simulink model "RT_IGBT"  (R2024b)
settings: Solver=ode4  StartTime=0.0  StopTime=2  FixedStep=Ts  RelTol=1e-3
PreLoadFcn:
  | Net_improve_init;L=Lac_MV;Tctrl=Ts;
PostLoadFcn:
  | Net_improve_init;L=Lac_MV;Tctrl=Ts;
InitFcn:
  | Net_improve_init;L=Lac_MV;Tctrl=Ts;
undefined symbols (not defined in the file): C1, dend, DiscIntNeverNeededParam, f_cari, fs, Lac_MV, numd, Pref, R1, Rac_MV, Ts, Vac_peak_MV, Vdc
libraries: powerlib_extras x5, spsControlledVoltageSourceLib x4, artemis x3, spsCurrentMeasurementLib x3, spsSeriesRLCBranchLib x3, spsVoltageMeasurementLib x3, rtlab x2, spsThreePhaseVIMeasurementLib x2, spsGroundLib x2, spsUniversalBridgeLib x1, spsIdealSwitchLib x1, spsPower3phInstantaneousLib x1
Description:
  | The Model initialization function Callback automatically
  | 
  | sets the sample time  to 2e-6 sec.  and loads the initial
  | 
  | states vector xInitial. The initial state vector is saved in the
  | 
  | power_acdrive_init.mat file.
  | 
  | 
  | 
  | Check  the Initial state checkbox in the Simulation
  | 
  | parameters/Workspace I/O to start in steady state with a
  | 
  | speed of 120 rad/s and a torque of 0 N.m/s,
  | 
  | 
  | Copyright 2008-2015 The MathWorks, Inc.
settings Model: Creator=WeiLi  LastModifiedBy=KeXing
settings SolverCC: AlgebraicLoopSolver=TrustRegion
settings DataIOCC: SaveFinalState=on  SaveFormat=Array  SignalLoggingSaveFormat=ModelDataLogs  SaveOutput=off  SaveTime=off  ReturnWorkspaceOutputs=off  SignalLoggingName=sigsOut
settings OptimizationCC: BlockReduction=off  ExpressionDepthLimit=2147483647  InitFltsAndDblsToZero=on  LifeSpan=inf
settings DebuggingCC: SaveWithParameterizedLinksMsg=none  UnderspecifiedInitializationDetection=Classic  MergeDetectMultiDrivingBlocksExec=none  CheckExecutionContextPreStartOutputMsg=on  SignalResolutionControl=TryResolveAllWithWarning  MultiTaskDSMMsg=warning  MultiTaskCondExecSysMsg=none  FcnCallInpInsideContextMsg=warning  UnconnectedInputMsg=warning  UnconnectedLineMsg=warning  StateNameClashWarn=warning  SFUnexpectedBacktrackingDiag=warning  SFNoUnconditionalDefaultTransitionDiag=warning  SFExecutionAtInitializationDiag=none  ArithmeticOperatorsInVariantConditions=warning
settings HardwareCC: ProdBitPerPointer=32  ProdBitPerSizeT=32  ProdBitPerPtrDiffT=32  ProdLargestAtomicFloat=None  ProdIntDivRoundTo=Undefined  ProdEndianess=Unspecified  ProdWordSize=32  ProdHWDeviceType=32-bit Generic  TargetUnknown=on
settings ModelReferenceCC: EnableRefExpFcnMdlSchedulingChecks=on  PropagateSignalLabelsOutOfModel=off
settings SFSimCC: SimUseLocalCustomCode=off  CustomCodeUndefinedFunction=UseInterfaceOnly
settings RTWCC: RTWUseLocalCustomCode=off  GPUComputeCapability=3.5
settings CodeAppCC: StateflowObjectComments=on
settings GRTTargetCC: TargetFcnLib=ansi_tfl_tmw.mat  TargetLangStandard=C89/C90 (ANSI)  CombineOutputUpdateFcns=off  GRTInterface=on
settings ConfigComp: CovMetricSettings=dw  CovSaveCumulativeToWorkspaceVar=on  CovSaveSingleToWorkspaceVar=on  CovExternalEMLEnable=off
settings SimscapeCC: SimscapeNormalizeSystem=off

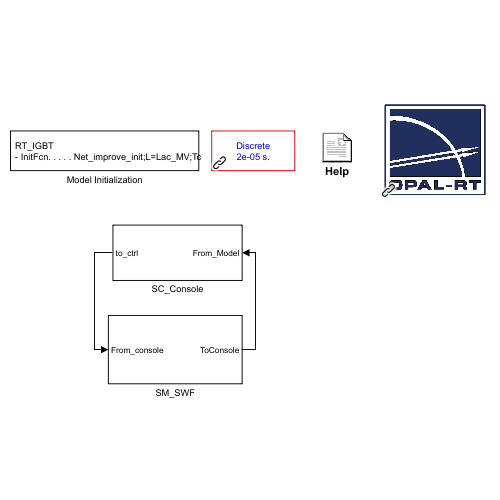
[thumbnail: Simulink's stored preview of the top-level diagram]
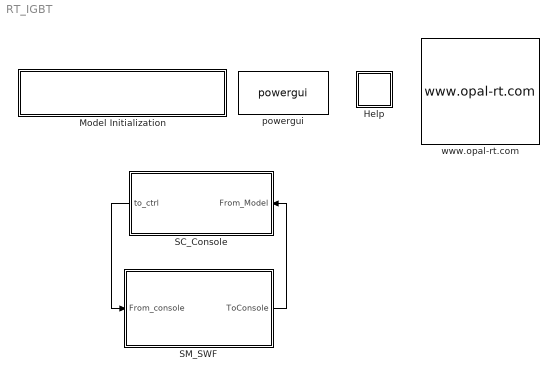
== system RT_IGBT ==
  Help : Subsystem  mask(OpDoc){docfile=../Help/help.html}
      mask init:
      | %patch([1,1,0,0,.8,1],[.8,0,0,1,1,.8],[.8 .8 .8]);
      | %patch([.15 .78 .78 .15 .15],[.8 .8 .83 .83 .8],[.9 .9 .9]);
      | %patch([.15 .78 .78 .15 .15],[.7 .7 .73 .73 .8],[.9 .9 .9]);
      | %patch([.15 .78 .78 .15 .15],[.6 .6 .63 .63 .6],[.9 .9 .9]);
      | %patch([.15 .78 .78 .15 .15],[.5 .5 .53 .53 .5],[.9 .9 .9]);
      | %patch([.15 .78 .78 .15 .15],[.4 .4 .43 .43 .4],[.9 .9 .9]);
      settings: OpenFcn=OpHelp_cb(gcb);
      mask Display: image(imread('opdoc.bmp'))
  Model Initialization : Subsystem  mask(Model Functions){InitFcnX=Net_improve_init;L=Lac_MV;Tctrl=Ts;, prel=on, posl=on, inif=on, strf=off}
      mask prompts: InitFcnX "Initialisation"; prel "Preload Function"; posl "PostLoad Function"; inif "InitFcn"; strf "StartFcn"
      mask init:
      | currentBlock = gcb;
      | root = bdroot(currentBlock);
      | 
      | if ~strcmp(get_param(root,'BlockDiagramType'),'library')
      |     if prel==1
      |         set_param(root, 'PreLoadFcn', InitFcnX);
      |     else
      |         set_param(root, 'PreLoadFcn', '');
      |     end
      |     if inif==1
      |         set_param(root, 'InitFcn', InitFcnX);
      |     else
      |         set_param(root, 'InitFcn', '');
      |     end
      |     if strf==1
      |         set_param(root, 'StartFcn', InitFcnX);
      |     else
      |         set_param(root, 'StartFcn', '');
      |     end
      |     if posl==1
      |         set_param(root, 'PostLoadFcn', InitFcnX);
      |     else
      |         set_param(root, 'PostLoadFcn', '');
      |     end
      | end
      | 
      | pos = get_param(currentBlock, 'Position');
      | width = pos(3) - pos(1); height = pos(4) - pos(2);
      | txt = [ upper(root) '\n' '- InitFcn. . . . . '  get_param(root, 'InitFcn') ];
      settings: CopyFcn=set_param(gcb,'LinkStatus','none')
      mask Display: text(5, height*0.5, txt, 'horizontalAlignment', 'left', 'verticalAlignment', 'middle') ;
  SC_Console : Subsystem
  SM_SWF : Subsystem
  powergui : spspowerguiLib/powergui  Priority=2  SimulationMode=Discrete  SampleTime=Ts  frequency=60  Iterations=50  frequencyindice=0  Pbase=100e6  ErrMax=1e-4  UnitsV=kV  UnitsW=MW  buscounter=0  FunctionMessages=off  echomessages=off  EnableUseOfTLC=off  CurrentSourceSwitches=off  DisableSnubberDevices=off  DisableRonSwitches=off  DisableVfSwitches=off  DisplayEquations=off  AutomaticDiscreteSolvers=off  SolverType=Backward Euler  Interpol=off  ExternalGateDelay=off  methode=off  Ts=0  x0status=blocks  SPID=off  SwTol=0  HookPort=off  NonlinearTolerance=1e-4  nMaxIteration=100  ContinueOnMaxIteration=off  RestoreLinks=warning  ResistiveCurrentMeasurement=off  Frange=[0:2:500]  Ylog=off  Xlog=on  ShowGrid=off  save=off  variable=ZData  structure=VI  ZoomFFT=off  StartTime=9  cycles=10  DisplayStyle=2  fundamental=300/pi  FreqAxis=off  MaxFrequency=1000  frequencyindicesteady=1  RmsSteady=1  display=off
  www.opal-rt.com : artemis/Internal/www.opal-rt.com  SystemSampleTime=-1  VariantActivationTime=update diagram  AllowFlexibleInterface=on  Latency=0  AutoFrameSizeCalculation=off
      settings: SourceProductName=Artemis
  wires:
  SM_SWF/1(ToConsole) -> SC_Console/1(From_Model)
  SC_Console/1(to_ctrl) -> SM_SWF/1(From_console)

== system RT_IGBT/Help ==

== system RT_IGBT/Model Initialization ==

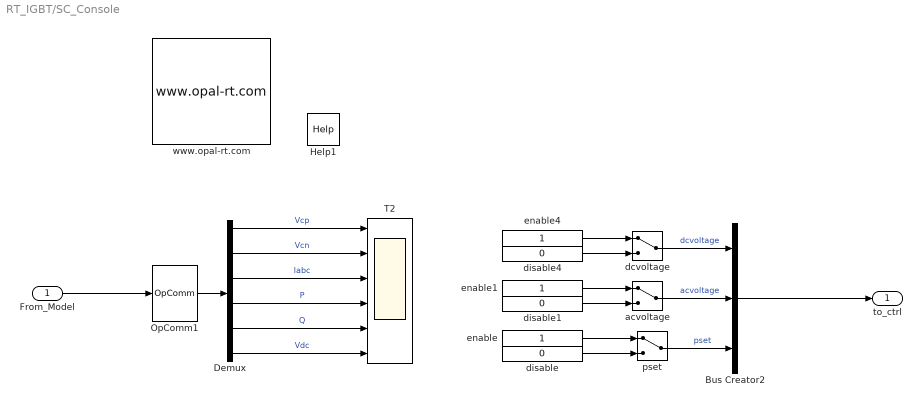
== system RT_IGBT/SC_Console ==
  From_Model : Inport
  Bus Creator2 : BusCreator  Inputs=3
  Demux : Demux  Outputs=6
  Help1 : artemis/Internal/Help  docfile=../help/help.html
      settings: SourceProductName=Artemis
  OpComm1 : rtlab/OpComm  nbport=1  groupe_acq=1  subsys_rate=Ts  st=0  Synchronization=off  Interpolation=on  Threshold=1.0  Missed_Data=off  Sim_Time=off  Samples=off  dynSigOut=off  from_console=0  warning_done=off  writeOpCommFile=off  Offset=off
      settings: SourceProductName=RT-LAB
  T2 : Scope  NumInputPorts=6
  acvoltage : ManualSwitch
  dcvoltage : ManualSwitch
  disable : Constant  Value=0
  disable1 : Constant  Value=0
  disable4 : Constant  Value=0
  enable : Constant
  enable1 : Constant
  enable4 : Constant
  pset : ManualSwitch
  www.opal-rt.com : artemis/Internal/www.opal-rt.com  SystemSampleTime=-1  VariantActivationTime=update diagram  AllowFlexibleInterface=on  Latency=0  AutoFrameSizeCalculation=off
      settings: SourceProductName=Artemis
  to_ctrl : Outport
  wires:
  enable/1 -> pset/1
  Demux/2 -> T2/2  "Vcn"
  OpComm1/1 -> Demux/1
  Bus Creator2/1 -> to_ctrl/1
  From_Model/1 -> OpComm1/1
  Demux/4 -> T2/4  "P"
  Demux/1 -> T2/1  "Vcp"
  acvoltage/1 -> Bus Creator2/2  "acvoltage"
  disable1/1 -> acvoltage/2
  disable/1 -> pset/2
  enable1/1 -> acvoltage/1
  Demux/3 -> T2/3  "Iabc"
  disable4/1 -> dcvoltage/2
  enable4/1 -> dcvoltage/1
  dcvoltage/1 -> Bus Creator2/1  "dcvoltage"
  pset/1 -> Bus Creator2/3  "pset"
  Demux/5 -> T2/5  "Q"
  Demux/6 -> T2/6  "Vdc"

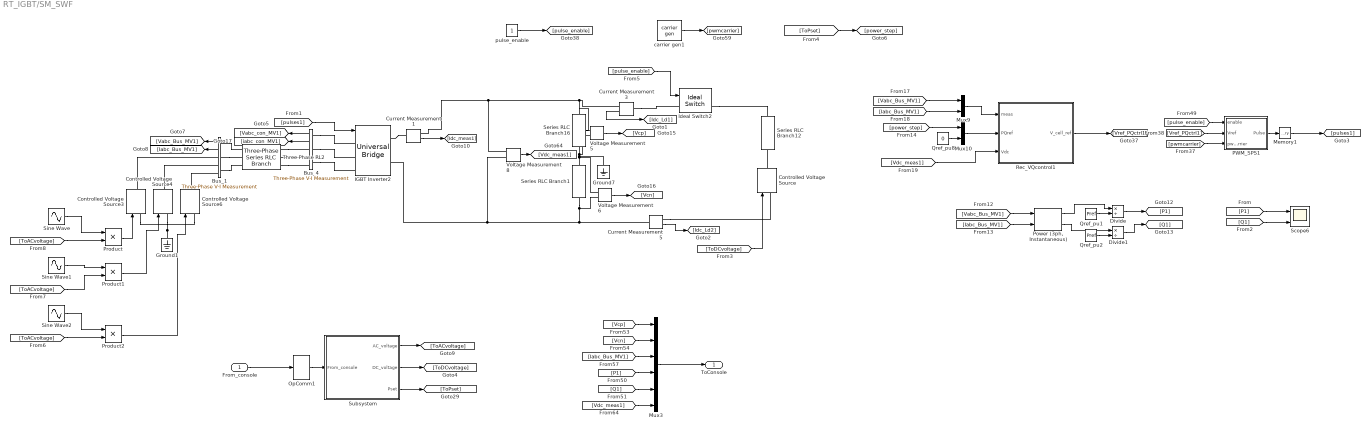
== system RT_IGBT/SM_SWF ==
  From_console : Inport
  Bus_1 : spsThreePhaseVIMeasurementLib/Three-Phase V-I Measurement  VoltageMeasurement=phase-to-ground  SetLabelV=off  LabelV=Vabc  Vpu=off  VpuLL=off  CurrentMeasurement=yes  SetLabelI=off  LabelI=Iabc  Ipu=off  Pbase=P_AC  Vbase=V_AC_prim  OutputType=Complex  PhasorSimulation=off  PSBequivalent=0
  Bus_4 : spsThreePhaseVIMeasurementLib/Three-Phase V-I Measurement  VoltageMeasurement=phase-to-ground  SetLabelV=off  LabelV=Vabc  Vpu=off  VpuLL=off  CurrentMeasurement=yes  SetLabelI=off  LabelI=Iabc  Ipu=off  Pbase=P_AC  Vbase=V_AC_prim  OutputType=Complex  PhasorSimulation=off  PSBequivalent=0
  Controlled Voltage Source : spsControlledVoltageSourceLib/Controlled Voltage Source  Initialize=on  Source_Type=DC  Amplitude=3000  Phase=0  Frequency=0  Measurements=None
  Controlled Voltage Source3 : spsControlledVoltageSourceLib/Controlled Voltage Source  Initialize=off  Source_Type=AC  Amplitude=0  Phase=0  Frequency=fs  Measurements=None
  Controlled Voltage Source4 : spsControlledVoltageSourceLib/Controlled Voltage Source  Initialize=off  Source_Type=AC  Amplitude=0  Phase=0  Frequency=fs  Measurements=None
  Controlled Voltage Source6 : spsControlledVoltageSourceLib/Controlled Voltage Source  Initialize=off  Source_Type=AC  Amplitude=0  Phase=0  Frequency=fs  Measurements=None
  Current Measurement1 : spsCurrentMeasurementLib/Current Measurement  PhasorSimulation=off  OutputType=Complex  PSBequivalent=0
  Current Measurement3 : spsCurrentMeasurementLib/Current Measurement  PhasorSimulation=off  OutputType=Complex  PSBequivalent=0
  Current Measurement5 : spsCurrentMeasurementLib/Current Measurement  PhasorSimulation=off  OutputType=Complex  PSBequivalent=0
  Divide : Product  Inputs=*/
  Divide1 : Product  Inputs=*/
  Ground1 : spsGroundLib/Ground  LConnTagsString=a
  Ground7 : spsGroundLib/Ground  LConnTagsString=a
  IGBT Inverter2 : spsUniversalBridgeLib/Universal Bridge  Arms=3  SnubberResistance=IGBT_Rs  SnubberCapacitance=1e-6  Device=IGBT / Diodes  Ron=IGBT_Ron  Lon=0  ForwardVoltages=[0 0]  ForwardVoltage=.8  GTOparameters=[ 1e-6 , 1e-6 ]  IGBTparameters=[0 0]  Measurements=Device voltages  Measurements_2=None  converterType=Rectifier
      settings: AttributesFormatString=\n
  Ideal Switch2 : spsIdealSwitchLib/Ideal Switch  Ron=0.001  Lon=0  IC=0  Rs=1e9  Cs=inf  Measurements=on
  Memory1 : Memory
  Mux10 : Mux  Inputs=2
  Mux3 : Mux  Inputs=6
  Mux9 : Mux  Inputs=2
  OpComm1 : rtlab/OpComm  nbport=1  groupe_acq=1  subsys_rate=Ts  st=0  Synchronization=on  Interpolation=on  Threshold=1.0  Missed_Data=off  Sim_Time=off  Samples=off  dynSigOut=off  from_console=1  warning_done=off  writeOpCommFile=off  Offset=off
      settings: SourceProductName=RT-LAB
  PWM_SPS1 : Subsystem
  "Power (3ph, Instantaneous)" : spsPower3phInstantaneousLib/Power (3ph, Instantaneous)
  Product : Product
  Product1 : Product
  Product2 : Product
  Qref_pu1 : Constant  Value=Pref
  Qref_pu2 : Constant  Value=Pref
  Qref_pu8 : Constant  Value=0
  Rec_VQcontrol1 : Subsystem  mask(converter controller){cm=off, base=[Pref, Vac_peak_MV*sqrt(3/2), Vdc/2, fs], LRx=[Lac_MV, Rac_MV], LRx_inpu=off, Kd=[0.3  2]*10/6  %was [1 0.1]   ; [0.1  1]*1, Kp=[0.3 1]*1     %was [1 0.1]   ; [0.1  1]*1, Kvdc=[2 10]*1;   %was [0.5 1]*20 for Cdc=320uF, Vabc_lim=[-1 1], limitVdq=1.1, nadv=6, xtrIctrl1=[0.4 10 10 -10], Ts=Tctrl}
      mask prompts: cm "control mode (check VQ/uncheck PQ), only one terminal in VQ mode"; base "base value for power(VA), ac voltage(V), dc voltage to ground(V), and frequenvy(Hz) [Sb, Vb, Vdcb,freq]"; LRx "commutation inductance and resistance [Lx, Rx]"; LRx_inpu "[Lx, Rx] in pu if checked/ SI unchecked"; Kd "Kp Ki for d-axis PI control [kp ki]"; Kp "Kp Ki for q-axis PI control [kp ki]"; Kvdc "Kp Ki for Vdc PI control [kp ki]"; Vabc_lim "output Vabc limit [min max]"; limitVdq "limit for Vd,Vq (pu, default = 1.1)"; nadv "nb of time step to compesate for delay (default=1)"; xtrIctrl1 "[kp, kp, limitmax, limitmin] for current control (default=[0.4, 10, 10, -10])"
      mask help:
      | input 1, 6 dimentions, Vabc, Iabc, (SI)
      | input 2, 2 dimentions, Pref, Qref (PU)
      | input 3, 6 dimentions, Vcap at up arm a, lower arm a, up arm b, lower arm b, up arm c and lower arm c.
      | input 4, 1 dimention, pulse on
      | input 5, 1 dimention
      |
      | power or current directions: to go into grid is positive
      mask init:
      | if cm==0;
      |     x=['PQ\nmode'];
      | else
      |     x=['VQ\nmode'];
      | end
      | 
      | Sb=base(1);            %VA 3phase power base;
      | Vb=base(2);       %V, line-line rms voltage base
      | Ib=Sb/(sqrt(3)*Vb); %A, rms current base
      | Zb=Vb^2/Sb ;        %ohm, impedence base
      | Vdc=base(3);      %V Vdc+ to ground or ground to Vdc- 
      | frq=base(4);
      | 
      | if LRx_inpu
      |     Rxpu=LRx(2);
      |     Lxpu=LRx(1);
      | else
      |     Rxpu=LRx(2)/Zb;
      |     Lxpu=LRx(1)*2*pi*frq/Zb;
      | end;
      | 
      | ks=Vdc*sqrt(3/2)/Vb;     % ma=1/ks for 1pu dc ->1pu ac;
      | 
      | Kp=Kd;
      mask DialogControl ParameterTabVar0 Prompt: parameters
      mask DialogControl ParameterTabVar01 Prompt: advanced
      mask Display: disp (x);
  Scope6 : Scope  NumInputPorts=2
  Series RLC Branch1 : spsSeriesRLCBranchLib/Series RLC Branch  LConnTagsString=__new0  RConnTagsString=__new0  BranchType=C  Resistance=R1  Inductance=1e-3  SetiL0=off  InitialCurrent=0  Capacitance=C1  Setx0=off  InitialVoltage=0  Measurements=None
  Series RLC Branch12 : spsSeriesRLCBranchLib/Series RLC Branch  LConnTagsString=__new0  RConnTagsString=__new0  BranchType=R  Resistance=3e3^2/(Pref)/10*2  Inductance=1e-3  SetiL0=off  InitialCurrent=0  Capacitance=C1  Setx0=off  InitialVoltage=0  Measurements=None
  Series RLC Branch16 : spsSeriesRLCBranchLib/Series RLC Branch  LConnTagsString=__new0  RConnTagsString=__new0  BranchType=C  Resistance=R1  Inductance=1e-3  SetiL0=off  InitialCurrent=0  Capacitance=C1  Setx0=off  InitialVoltage=0  Measurements=None
  Sine Wave : Sin  Amplitude=3e3/2*sqrt(2/3)  Frequency=2*pi*fs  SampleTime=0
  Sine Wave1 : Sin  Amplitude=3e3/2*sqrt(2/3)  Frequency=2*pi*fs  Phase=-2*pi/3  SampleTime=0
  Sine Wave2 : Sin  Amplitude=3e3/2*sqrt(2/3)  Frequency=2*pi*fs  Phase=+2*pi/3  SampleTime=0
  Subsystem : Subsystem
  Three-Phase RL2 : spsThreePhaseSeriesRLCBranchLib/Three-Phase Series RLC Branch  LConnTagsString=A|B|C  RConnTagsString=A|B|C  BranchType=RL  Resistance=Rac_MV  Inductance=Lac_MV  Capacitance=1e-6  Measurements=None
  Voltage Measurement5 : spsVoltageMeasurementLib/Voltage Measurement  PhasorSimulation=off  OutputType=Complex  PSBequivalent=0
  Voltage Measurement6 : spsVoltageMeasurementLib/Voltage Measurement  PhasorSimulation=off  OutputType=Complex  PSBequivalent=0
  Voltage Measurement8 : spsVoltageMeasurementLib/Voltage Measurement  PhasorSimulation=off  OutputType=Complex  PSBequivalent=0
  carrier gen1 : libMMCcpuv2/carrier gen  fc=f_cari*2  range=[ 1 -1]  Ms=3  Ns=1
  pulse_enable : Constant
  ToConsole : Outport
  wires:
  Bus_1/1 -> [Vabc_Bus_MV1]
  Subsystem/2(DC_voltage) -> [ToDCvoltage]
  Sine Wave1/1 -> Product1/1
  Bus_1/2 -> [Iabc_Bus_MV1]
  [Q1] -> Scope6/2
  Qref_pu2/1 -> Divide1/2
  From_console/1 -> OpComm1/1
  Product/1 -> Controlled Voltage Source3/1
  [pwmcarrier] -> PWM_SPS1/3(pwmcarrier)
  Bus_4/1 -> [Vabc_con_MV1]
  [pulse_enable] -> Ideal Switch2/1
  Mux3/1 -> ToConsole/1
  Divide1/1 -> [Q1]
  Voltage Measurement5/1 -> [Vcp]
  [Vabc_Bus_MV1] -> Mux9/1
  [P1] -> Mux3/4
  [Vcn] -> Mux3/2
  [pulses1] -> IGBT Inverter2/1
  Current Measurement5/1 -> [Idc_Ld2]
  Mux10/1 -> Rec_VQcontrol1/2(PQref)
  Sine Wave2/1 -> Product2/1
  [Q1] -> Mux3/5
  Bus_4/2 -> [iabc_con_MV1]
  Mux9/1 -> Rec_VQcontrol1/1(meas)
  OpComm1/1 -> Subsystem/1(From_console)
  [ToPset] -> [power_step]
  [ToACvoltage] -> Product/2
  Qref_pu8/1 -> Mux10/2
  Product2/1 -> Controlled Voltage Source6/1
  Subsystem/3(Pset) -> [ToPset]
  [power_step] -> Mux10/1
  pulse_enable/1 -> [pulse_enable]
  [Iabc_Bus_MV1] -> "Power (3ph, Instantaneous)"/2
  [ToDCvoltage] -> Controlled Voltage Source/1
  Current Measurement3/1 -> [Idc_Ld1]
  "Power (3ph, Instantaneous)"/2 -> Divide1/1
  Sine Wave/1 -> Product/1
  "Power (3ph, Instantaneous)"/1 -> Divide/1
  PWM_SPS1/1(Pulse) -> Memory1/1
  [Iabc_Bus_MV1] -> Mux9/2
  [Vabc_Bus_MV1] -> "Power (3ph, Instantaneous)"/1
  Voltage Measurement6/1 -> [Vcn]
  [Vdc_meas1] -> Mux3/6
  Qref_pu1/1 -> Divide/2
  Divide/1 -> [P1]
  Voltage Measurement8/1 -> [Vdc_meas1]
  [Vdc_meas1] -> Rec_VQcontrol1/3(Vdc)
  Memory1/1 -> [pulses1]
  [Vref_PQctrl1] -> PWM_SPS1/2(Vref)
  [Iabc_Bus_MV1] -> Mux3/3
  carrier gen1/1 -> [pwmcarrier]
  Rec_VQcontrol1/1(V_cell_ref) -> [Vref_PQctrl1]
  [P1] -> Scope6/1
  Current Measurement1/1 -> [Idc_meas1]
  [Vcp] -> Mux3/1
  Product1/1 -> Controlled Voltage Source4/1
  [pulse_enable] -> PWM_SPS1/1(enable)
  [ToACvoltage] -> Product2/2
  Subsystem/1(AC_voltage) -> [ToACvoltage]
  [ToACvoltage] -> Product1/2
  connections:
  Series RLC Branch1/LConn1 -- Voltage Measurement6/LConn1 -- Ground7/LConn1 -- Voltage Measurement5/LConn2 -- Series RLC Branch16/RConn1
  Controlled Voltage Source/RConn1 -- Series RLC Branch12/LConn1
  Bus_1/LConn2 -- Three-Phase RL2/LConn2
  Ground1/LConn1 -- Controlled Voltage Source6/LConn1 -- Controlled Voltage Source3/LConn1 -- Controlled Voltage Source4/LConn1
  Ideal Switch2/RConn1 -- Series RLC Branch12/RConn1
  Bus_4/LConn3 -- IGBT Inverter2/LConn3
  Series RLC Branch1/RConn1 -- Voltage Measurement6/LConn2 -- IGBT Inverter2/RConn2 -- Voltage Measurement8/LConn2 -- Current Measurement5/LConn1
  Three-Phase RL2/RConn1 -- Bus_4/RConn1
  Bus_1/LConn3 -- Three-Phase RL2/LConn3
  Voltage Measurement8/LConn1 -- Voltage Measurement5/LConn1 -- Series RLC Branch16/LConn1 -- Current Measurement3/RConn1 -- Current Measurement1/RConn1
  Current Measurement5/RConn1 -- Controlled Voltage Source/LConn1
  Three-Phase RL2/RConn3 -- Bus_4/RConn3
  Controlled Voltage Source4/RConn1 -- Bus_1/RConn2
  Bus_4/LConn2 -- IGBT Inverter2/LConn2
  Bus_1/LConn1 -- Three-Phase RL2/LConn1
  Current Measurement3/LConn1 -- Ideal Switch2/LConn1
  Three-Phase RL2/RConn2 -- Bus_4/RConn2
  Controlled Voltage Source3/RConn1 -- Bus_1/RConn1
  Current Measurement1/LConn1 -- IGBT Inverter2/RConn1
  Controlled Voltage Source6/RConn1 -- Bus_1/RConn3
  Bus_4/LConn1 -- IGBT Inverter2/LConn1

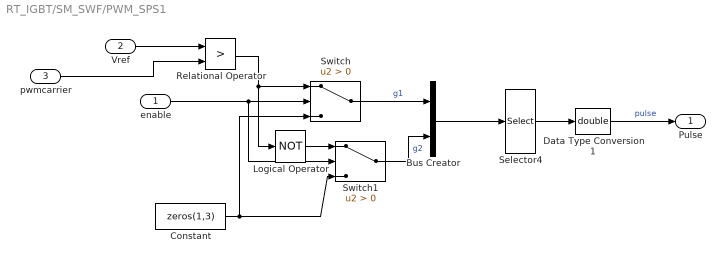
== system RT_IGBT/SM_SWF/PWM_SPS1 ==
  enable : Inport
  Vref : Inport  Port=2
  pwmcarrier : Inport  Port=3
  Bus Creator : BusCreator  Inputs=2
  Constant : Constant  Value=zeros(1,3)
  Data Type Conversion1 : DataTypeConversion  OutDataTypeStr=double  SaturateOnIntegerOverflow=off  RndMeth=Floor
  Logical Operator : Logic  Operator=NOT  AllPortsSameDT=off  OutDataTypeStr=boolean
  Relational Operator : RelationalOperator  Operator=>  OutDataTypeStr=boolean  InputSameDT=off
  Selector4 : Selector  InputPortWidth=6  IndexOptions=Index vector (dialog)  Indices=[1 4 2 5 3 6]  OutputSizes=1
  Switch : Switch  Criteria=u2 > Threshold  SaturateOnIntegerOverflow=off  InputSameDT=off
  Switch1 : Switch  Criteria=u2 > Threshold  SaturateOnIntegerOverflow=off  InputSameDT=off
  Pulse : Outport  VectorParamsAs1DForOutWhenUnconnected=off
  wires:
  Vref/1 -> Relational Operator/1
  pwmcarrier/1 -> Relational Operator/2
  enable/1 -> Switch1/2, Switch/2
  Relational Operator/1 -> Logical Operator/1, Switch/1
  Switch/1 -> Bus Creator/1  "g1"
  Switch1/1 -> Bus Creator/2  "g2"
  Logical Operator/1 -> Switch1/1
  Constant/1 -> Switch/3, Switch1/3
  Selector4/1 -> Data Type Conversion1/1
  Bus Creator/1 -> Selector4/1
  Data Type Conversion1/1 -> Pulse/1  "pulse"

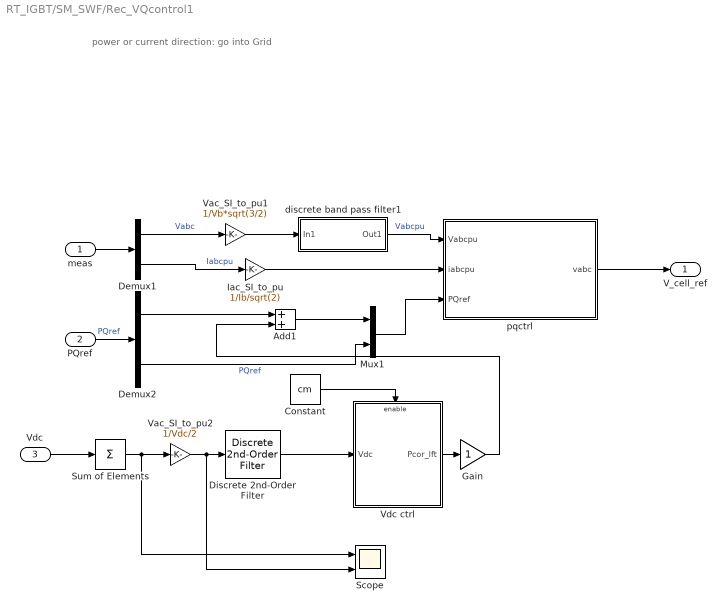
== system RT_IGBT/SM_SWF/Rec_VQcontrol1 ==
  note: power or current direction: go into Grid
  meas : Inport
  PQref : Inport  Port=2
  Vdc : Inport  Port=3
  Add1 : Sum
  Constant : Constant  Value=cm
  Demux1 : Demux  Outputs=[3 3 ]
  Demux2 : Demux  Outputs=2
  Discrete 2nd-Order Filter : powerlib_extras/Discrete  Control Blocks/Discrete  2nd-Order Filter  FilterType=Lowpass  Fo=90  Zeta=0.707  Ts=Ts  Initialize=off  Vac_Init=[0.8 -25 60]  Vdc_Init=-0.4  PlotResponse=off  param1=[1 500 1]
  Gain : Gain
  Iac_SI_to_pu : Gain  Gain=1/Ib/sqrt(2)
  Mux1 : Mux  Inputs=2
  Scope : Scope  NumInputPorts=2
  Sum of Elements : Sum  Inputs=+
  Vac_SI_to_pu1 : Gain  Gain=1/Vb*sqrt(3/2)
  Vac_SI_to_pu2 : Gain  Gain=1/Vdc/2  SampleTime=Ts
  Vdc ctrl : Subsystem
  discrete band pass filter1 : Subsystem  mask(discrete transfer Fcn generator){Fo=frq, adj1=1, inistate=0, Ts=Ts, bodedw=off}
      mask prompts: Fo "F0 (Hz)"; adj1 "adj (1 for no adjustment, larger adj for wider band pass)"; inistate "Initial states"; Ts "Sample time (must be explicite)"; bodedw "draw Bode diagram of filter"
      mask help:
      | This block transfer a continous TF to a discrete TF
      | using Bilinear (Tustin) approximation
      mask init:
      | AD1=tf([1 0],1);
      | 
      | %second order
      | % Fo=50; %cut off freq.
      | % omega0=Fo*2*pi;
      | % adj1=3;   %adjustment 1
      | Zeta= 0.707*adj1; %Damping factor Zeta ( Q = 1 / (2*Zeta) ):
      | Wo=2*pi*Fo;
      | % str=sprintf(' Fo=%iHz\n\n',Fo);
      |  n2=0; n1=0;n0=Wo*Wo;
      |  d2=1;d1=2*Zeta*Wo;d0=Wo*Wo;
      | numc=[n2 n1 n0];
      | denc=[d2 d1 d0];
      | AD3=tf(numc,denc);
      | 
      | AD4=AD1*AD3;
      | [mag1,pha1]=bode(AD4,Wo);
      | mag0=mag1;
      | AD=AD4/mag0;
      | 
      | if bodedw==1
      |     figure;
      |     h=bodeplot(AD1,AD3,AD);
      |     setoptions(h,'FreqUnits','Hz');
      |     grid on;
      |     title(['Bode Diagram, adj=',num2str(adj1)]);
      | end;
      |     
      | % gg=tf(num,den);
      | ggd=c2d(AD,Ts,'tustin');
      | [numd,dend] = tfdata(ggd,'v');
  pqctrl : Subsystem
  V_cell_ref : Outport  VectorParamsAs1DForOutWhenUnconnected=off
  wires:
  Constant/1 -> Vdc ctrl/Enable
  Vac_SI_to_pu1/1 -> discrete band pass filter1/1(In1)
  Vac_SI_to_pu2/1 -> Scope/2, Discrete 2nd-Order Filter/1
  Vdc/1 -> Sum of Elements/1
  Discrete 2nd-Order Filter/1 -> Vdc ctrl/1(Vdc)
  Mux1/1 -> pqctrl/3(PQref)
  Demux2/2 -> Mux1/2  "PQref"
  Add1/1 -> Mux1/1
  Vdc ctrl/1(Pcor_lft) -> Gain/1
  Demux2/1 -> Add1/1
  Iac_SI_to_pu/1 -> pqctrl/2(iabcpu)
  Demux1/1 -> Vac_SI_to_pu1/1  "Vabc"
  Demux1/2 -> Iac_SI_to_pu/1  "Iabcpu"
  meas/1 -> Demux1/1
  discrete band pass filter1/1(Out1) -> pqctrl/1(Vabcpu)  "Vabcpu"
  PQref/1 -> Demux2/1  "PQref"
  pqctrl/1(vabc) -> V_cell_ref/1
  Sum of Elements/1 -> Scope/1, Vac_SI_to_pu2/1
  Gain/1 -> Add1/2

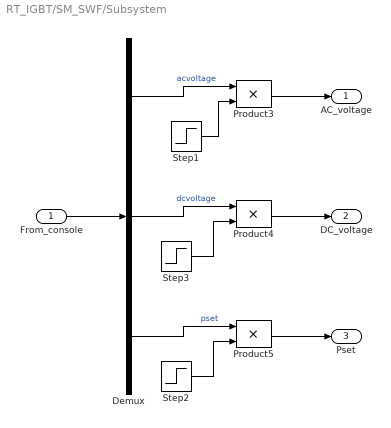
== system RT_IGBT/SM_SWF/Subsystem ==
  From_console : Inport
  Demux : Demux  Outputs=3
  Product3 : Product  RndMeth=Zero
  Product4 : Product  RndMeth=Zero
  Product5 : Product  RndMeth=Zero
  Step1 : Step  Time=2.0  Before=1.0  After=0.8  SampleTime=0
  Step2 : Step  Time=1.0  Before=-0.8  After=-0.6  SampleTime=0
  Step3 : Step  Time=2.0  Before=3000  After=2800  SampleTime=0
  AC_voltage : Outport
  DC_voltage : Outport  Port=2
  Pset : Outport  Port=3
  wires:
  Product3/1 -> AC_voltage/1
  Product5/1 -> Pset/1
  Demux/3 -> Product5/1  "pset"
  Demux/2 -> Product4/1  "dcvoltage"
  Product4/1 -> DC_voltage/1
  Step2/1 -> Product5/2
  Step3/1 -> Product4/2
  Step1/1 -> Product3/2
  Demux/1 -> Product3/1  "acvoltage"
  From_console/1 -> Demux/1

== system RT_IGBT/SM_SWF/Rec_VQcontrol1/Vdc ctrl ==
  Vdc : Inport
  Enable : EnablePort  StatesWhenEnabling=reset
  Vdc_ctrler1 : Subsystem
  Pcor_lft : Outport  OutputWhenDisabled=reset  InitialOutput=0  VectorParamsAs1DForOutWhenUnconnected=off
  wires:
  Vdc_ctrler1/1(delP) -> Pcor_lft/1  "Pclft"
  Vdc/1 -> Vdc_ctrler1/1(Vcap)

== system RT_IGBT/SM_SWF/Rec_VQcontrol1/discrete band pass filter1 ==
  In1 : Inport
  Discrete Transfer Fcn : DiscreteTransferFcn  Numerator=numd  Denominator=dend  InitialStates=inistate  SampleTime=Ts
  Out1 : Outport  VectorParamsAs1DForOutWhenUnconnected=off
  wires:
  Discrete Transfer Fcn/1 -> Out1/1
  In1/1 -> Discrete Transfer Fcn/1

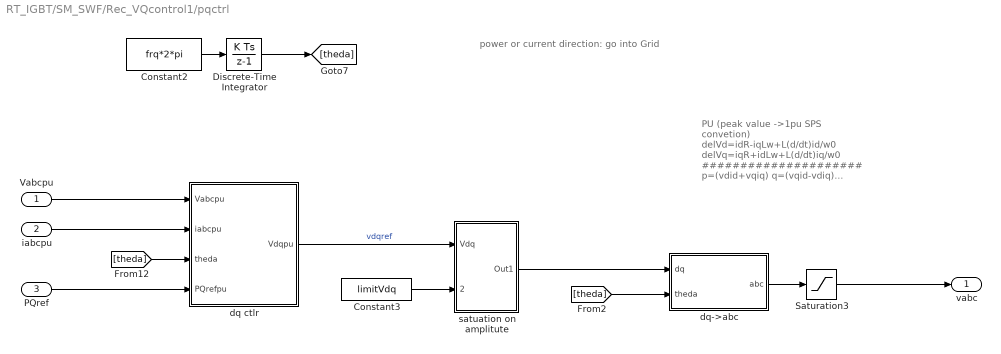
== system RT_IGBT/SM_SWF/Rec_VQcontrol1/pqctrl ==
  note: PU
      | (peak value ->1pu
      | SPS convetion)
      |
      | delVd=idR-iqLw+L(d/dt)id/w0
      | delVq=iqR+idLw+L(d/dt)iq/w0
      | #####################
      | p=(vdid+vqiq)
      | q=(vqid-vdiq)
      | =>
      | Id=(Vd*P+Vq*Q)/C
      | Iq=(Vq*P-Vd*Q)/C
      | C=Vd^2+Vq^2
  note: power or current direction: go into Grid
  Vabcpu : Inport
  iabcpu : Inport  Port=2
  PQref : Inport  Port=3
  Constant2 : Constant  Value=frq*2*pi
  Constant3 : Constant  Value=limitVdq
  Discrete-Time Integrator : DiscreteIntegrator  SampleTime=Ts  ICPrevOutput=DiscIntNeverNeededParam  ICPrevScaledInput=DiscIntNeverNeededParam
  Saturation3 : Saturate  UpperLimit=Vabc_lim(2)  LowerLimit=Vabc_lim(1)
  dq ctlr : Subsystem
  dq->abc : Subsystem
  "satuation on amplitute " : Subsystem
  vabc : Outport  VectorParamsAs1DForOutWhenUnconnected=off
  wires:
  Saturation3/1 -> vabc/1
  [theda] -> dq->abc/2(theda)
  dq->abc/1(abc) -> Saturation3/1
  Constant3/1 -> "satuation on amplitute "/2(limitVdq)
  "satuation on amplitute "/1(Out1) -> dq->abc/1(dq)
  Constant2/1 -> Discrete-Time Integrator/1
  Discrete-Time Integrator/1 -> [theda]
  [theda] -> dq ctlr/3(theda)
  dq ctlr/1(Vdqpu) -> "satuation on amplitute "/1(Vdq)  "vdqref"
  Vabcpu/1 -> dq ctlr/1(Vabcpu)
  iabcpu/1 -> dq ctlr/2(iabcpu)
  PQref/1 -> dq ctlr/4(PQrefpu)

== system RT_IGBT/SM_SWF/Rec_VQcontrol1/Vdc ctrl/Vdc_ctrler1 ==
  Vcap : Inport
  Add2 : Sum  Inputs=+-
  PI_d2 : Subsystem  AncestorBlock=|  DialogController=POWERSYS.PowerSysDialog  mask(Discrete PI Controller){Kp=Kvdc(1), Ki=Kvdc(2), Par_Limits=[1 -1]*1, Init=0, Ts=Ts}
      | powerlib_extras/Discrete 
      | Control Blocks/Discrete
      | PI Controller
      mask prompts: Kp "Proportional gain (Kp):"; Ki "Integral gain (Ki):"; Par_Limits "Output limits: [ Upper   Lower ]"; Init "Output initial value:"; Ts "Sample time:"
      mask help: This block implements a discrete PI controller.
      mask init:
      | UpperLimit=Par_Limits(1);
      | LowerLimit=Par_Limits(2);
      | power_initmask();
      mask Help: This block is part of a subset of blocks in the Extras library that does not have documentation associated with it, other than the block mask description.
      mask Display: disp('PI');
  Saturation : Saturate  UpperLimit=0.1  LowerLimit=-0.1
      settings: AttributesFormatString=%<LowerLimit>~%<UpperLimit>
  Vdcpuref : Constant
  Vdctrl : Scope  NumInputPorts=2
  delP : Outport  OutputWhenDisabled=reset  InitialOutput=[0]  VectorParamsAs1DForOutWhenUnconnected=off
  wires:
  PI_d2/1(Out) -> delP/1, Vdctrl/2  "PIVdc"
  Saturation/1 -> PI_d2/1(Error)
  Vdcpuref/1 -> Add2/2
  Vcap/1 -> Add2/1, Vdctrl/1
  Add2/1 -> Saturation/1  "delVdc"

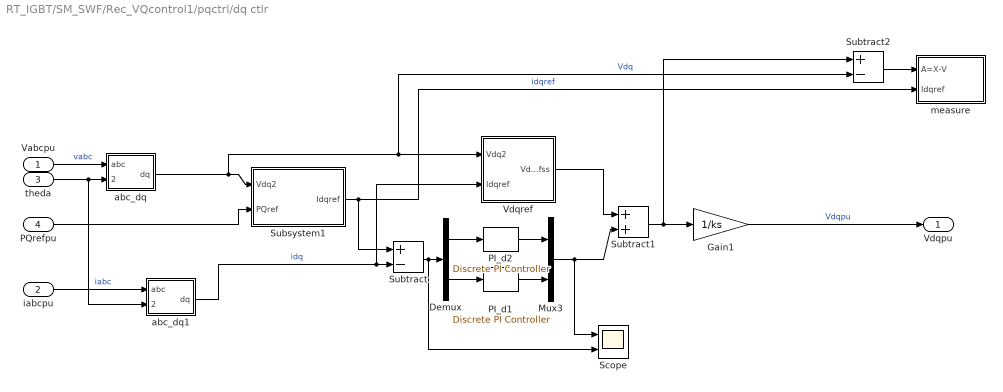
== system RT_IGBT/SM_SWF/Rec_VQcontrol1/pqctrl/dq ctlr ==
  Vabcpu : Inport
  iabcpu : Inport  Port=2
  theda : Inport  Port=3
  PQrefpu : Inport  Port=4
  Demux : Demux  Outputs=2
  Gain1 : Gain  Gain=1/ks
  Mux3 : Mux  Inputs=2
  PI_d1 : powerlib_extras/Discrete  Control Blocks/Discrete PI Controller  Kp=Kp(1)  Ki=Kp(2)  Par_Limits=[1 -1]*0.15  Init=0  Ts=Ts
  PI_d2 : powerlib_extras/Discrete  Control Blocks/Discrete PI Controller  Kp=Kd(1)  Ki=Kd(2)  Par_Limits=[1 -1]*0.25  Init=0  Ts=Ts
  Scope : Scope  NumInputPorts=2
  Subsystem1 : Subsystem
  Subtract : Sum  Inputs=+-
  Subtract1 : Sum
  Subtract2 : Sum  Inputs=+-
  Vdqref : Subsystem
  abc_dq : Subsystem
  abc_dq1 : Subsystem
  measure : Subsystem
  Vdqpu : Outport  VectorParamsAs1DForOutWhenUnconnected=off
  wires:
  Subtract2/1 -> measure/1(A=X-V)
  Subsystem1/1(Idqref) -> measure/2(Idqref), Subtract/1  "idqref"
  abc_dq/1(dq) -> Subtract2/2, Vdqref/1(Vdq2), Subsystem1/1(Vdq2)  "Vdq"
  abc_dq1/1(dq) -> Vdqref/2(Idqref), Subtract/2  "idq"
  Subtract/1 -> Scope/2, Demux/1
  Demux/1 -> PI_d2/1
  Demux/2 -> PI_d1/1
  Vdqref/1(Vdqrefss) -> Subtract1/1
  PI_d2/1 -> Mux3/1
  PI_d1/1 -> Mux3/2
  Mux3/1 -> Scope/1, Subtract1/2
  Subtract1/1 -> Subtract2/1, Gain1/1
  Vabcpu/1 -> abc_dq/1(abc)  "vabc"
  theda/1 -> abc_dq/2(theta), abc_dq1/2(theta)
  PQrefpu/1 -> Subsystem1/2(PQref)
  iabcpu/1 -> abc_dq1/1(abc)  "iabc"
  Gain1/1 -> Vdqpu/1  "Vdqpu"

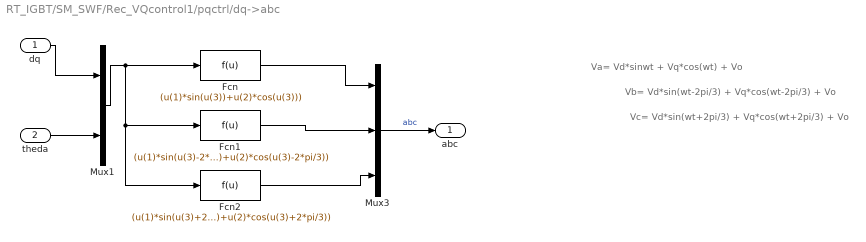
== system RT_IGBT/SM_SWF/Rec_VQcontrol1/pqctrl/dq->abc ==
  note: Va= Vd*sinwt + Vq*cos(wt) + Vo
  note: Vb= Vd*sin(wt-2pi/3) + Vq*cos(wt-2pi/3) + Vo
  note: Vc= Vd*sin(wt+2pi/3) + Vq*cos(wt+2pi/3) + Vo
  dq : Inport
  theda : Inport  Port=2
  Fcn : Fcn  Expr=(u(1)*sin(u(3))+u(2)*cos(u(3)))
  Fcn1 : Fcn  Expr=(u(1)*sin(u(3)-2*pi/3)+u(2)*cos(u(3)-2*pi/3))
  Fcn2 : Fcn  Expr=(u(1)*sin(u(3)+2*pi/3)+u(2)*cos(u(3)+2*pi/3))
  Mux1 : Mux  Inputs=2
  Mux3 : Mux  Inputs=3
  abc : Outport  VectorParamsAs1DForOutWhenUnconnected=off
  wires:
  Fcn2/1 -> Mux3/3
  Fcn1/1 -> Mux3/2
  Fcn/1 -> Mux3/1
  Mux1/1 -> Fcn/1, Fcn2/1, Fcn1/1
  dq/1 -> Mux1/1
  theda/1 -> Mux1/2
  Mux3/1 -> abc/1  "abc"

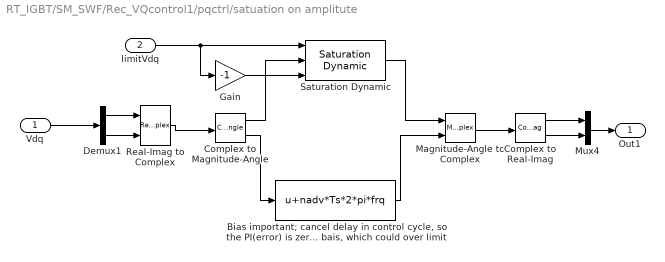
== system RT_IGBT/SM_SWF/Rec_VQcontrol1/pqctrl/satuation on amplitute  ==
  Vdq : Inport
  limitVdq : Inport  Port=2
  "Bias important; cancel delay in control cycle, so the PI(error) is zero, other wise PI(errer) is bais, which could over limit" : Bias  Bias=nadv*Ts*2*pi*frq  SaturateOnIntegerOverflow=off
  Complex to Magnitude-Angle : ComplexToMagnitudeAngle
  Complex to Real-Imag : ComplexToRealImag
  Demux1 : Demux  Outputs=2
  Gain : Gain  Gain=-1
  Magnitude-Angle to Complex : MagnitudeAngleToComplex
  Mux4 : Mux  Inputs=2
  Real-Imag to Complex : RealImagToComplex
  Saturation Dynamic : simulink/Discontinuities/Saturation Dynamic  OutMin=[]  OutMax=[]  OutDataTypeStr=Inherit: Same as second input  OutDataType=fixdt(1, 16)  OutScaling=2^-10  DoSatur=off
  Out1 : Outport  VectorParamsAs1DForOutWhenUnconnected=off
  wires:
  "Bias important; cancel delay in control cycle, so the PI(error) is zero, other wise PI(errer) is bais, which could over limit"/1 -> Magnitude-Angle to Complex/2
  Gain/1 -> Saturation Dynamic/3
  limitVdq/1 -> Saturation Dynamic/1, Gain/1
  Complex to Magnitude-Angle/1 -> Saturation Dynamic/2
  Saturation Dynamic/1 -> Magnitude-Angle to Complex/1
  Demux1/1 -> Real-Imag to Complex/1
  Demux1/2 -> Real-Imag to Complex/2
  Real-Imag to Complex/1 -> Complex to Magnitude-Angle/1
  Complex to Magnitude-Angle/2 -> "Bias important; cancel delay in control cycle, so the PI(error) is zero, other wise PI(errer) is bais, which could over limit"/1
  Magnitude-Angle to Complex/1 -> Complex to Real-Imag/1
  Complex to Real-Imag/2 -> Mux4/2
  Complex to Real-Imag/1 -> Mux4/1
  Mux4/1 -> Out1/1
  Vdq/1 -> Demux1/1

== system RT_IGBT/SM_SWF/Rec_VQcontrol1/Vdc ctrl/Vdc_ctrler1/PI_d2 ==
  note: Discrete PID Controller
  note: Pierre Giroux, Gilbert Sybille
      | Power System Simulation Laboratory
      | IREQ, Hydro-Quebc
  Error : Inport  SampleTime=Ts
  Discrete-Time Integrator : DiscreteIntegrator  InitialCondition=Init  SampleTime=Ts  LimitOutput=on  UpperSaturationLimit=UpperLimit  LowerSaturationLimit=LowerLimit  ICPrevOutput=DiscIntNeverNeededParam  ICPrevScaledInput=DiscIntNeverNeededParam
  Kp4 : Gain  Gain=Kp  SaturateOnIntegerOverflow=on  SampleTime=Ts  OutDataTypeStr=Inherit: Same as input  ParamDataTypeStr=Inherit: Same as input
  Kp5 : Gain  Gain=Ki  SaturateOnIntegerOverflow=on  SampleTime=Ts  OutDataTypeStr=Inherit: Same as input  ParamDataTypeStr=Inherit: Same as input
  Saturation2 : Saturate  UpperLimit=UpperLimit  LowerLimit=LowerLimit  SampleTime=Ts
  Sum6 : Sum  InputSameDT=on  SaturateOnIntegerOverflow=on  SampleTime=Ts  OutDataTypeStr=Inherit: Same as first input
  Zero-Order Hold : ZeroOrderHold  SampleTime=Ts
  Out : Outport  SampleTime=Ts  InitialOutput=0  VectorParamsAs1DForOutWhenUnconnected=off
  wires:
  Zero-Order Hold/1 -> Sum6/1  "prop"
  Saturation2/1 -> Out/1
  Discrete-Time Integrator/1 -> Sum6/2  "int"
  Kp4/1 -> Zero-Order Hold/1
  Kp5/1 -> Discrete-Time Integrator/1
  Sum6/1 -> Saturation2/1
  Error/1 -> Kp5/1, Kp4/1

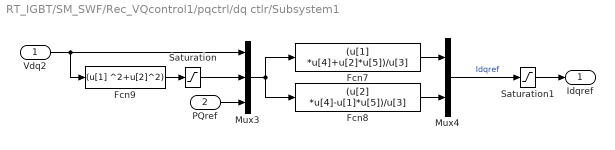
== system RT_IGBT/SM_SWF/Rec_VQcontrol1/pqctrl/dq ctlr/Subsystem1 ==
  Vdq2 : Inport
  PQref : Inport  Port=2
  Fcn7 : Fcn  Expr=(u[1] *u[4]+u[2]*u[5])/u[3]
  Fcn8 : Fcn  Expr=(u[2] *u[4]-u[1]*u[5])/u[3]
  Fcn9 : Fcn  Expr=(u[1] ^2+u[2]^2)
  Mux3 : Mux  Inputs=[2 1 2]
  Mux4 : Mux  Inputs=2
  Saturation : Saturate  UpperLimit=inf  LowerLimit=0.01
  Saturation1 : Saturate  UpperLimit=1.5  LowerLimit=-1.5
  Idqref : Outport  VectorParamsAs1DForOutWhenUnconnected=off
  wires:
  Saturation1/1 -> Idqref/1
  Vdq2/1 -> Fcn9/1, Mux3/1
  Mux3/1 -> Fcn8/1, Fcn7/1
  Fcn9/1 -> Saturation/1
  Fcn7/1 -> Mux4/1
  Fcn8/1 -> Mux4/2
  Mux4/1 -> Saturation1/1  "Idqref"
  PQref/1 -> Mux3/3
  Saturation/1 -> Mux3/2

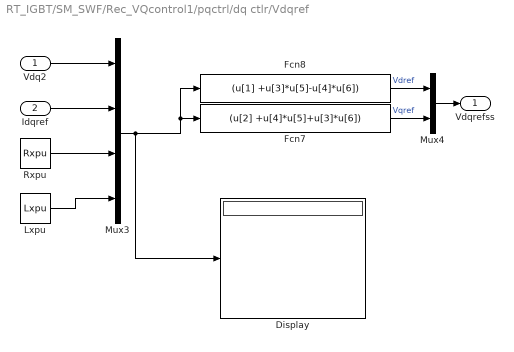
== system RT_IGBT/SM_SWF/Rec_VQcontrol1/pqctrl/dq ctlr/Vdqref ==
  Vdq2 : Inport
  Idqref : Inport  Port=2
  Display : Display
      settings: Decimation=50
  Fcn7 : Fcn  Expr=(u[2] +u[4]*u[5]+u[3]*u[6])
  Fcn8 : Fcn  Expr=(u[1] +u[3]*u[5]-u[4]*u[6])
  Lxpu : Constant  Value=Lxpu
  Mux3 : Mux
  Mux4 : Mux  Inputs=2
  Rxpu : Constant  Value=Rxpu
  Vdqrefss : Outport  VectorParamsAs1DForOutWhenUnconnected=off
  wires:
  Lxpu/1 -> Mux3/4
  Rxpu/1 -> Mux3/3
  Mux3/1 -> Display/1, Fcn8/1, Fcn7/1
  Fcn8/1 -> Mux4/1  "Vdref"
  Fcn7/1 -> Mux4/2  "Vqref"
  Vdq2/1 -> Mux3/1
  Idqref/1 -> Mux3/2
  Mux4/1 -> Vdqrefss/1

== system RT_IGBT/SM_SWF/Rec_VQcontrol1/pqctrl/dq ctlr/abc_dq ==
  abc : Inport
  theta : Inport  Port=2
  Mux2 : Mux  Inputs=2
  Selector3 : Selector  InputPortWidth=3  IndexOptions=Index vector (dialog)  Indices=[1 2]  OutputSizes=1
  Trigonometric Function2 : Trigonometry
  Trigonometric Function3 : Trigonometry  Operator=cos
  abc/dq1 : powerlib_extras/Measurements/abc_to_dq0 Transformation
  dq : Outport  VectorParamsAs1DForOutWhenUnconnected=off
  wires:
  abc/1 -> abc/dq1/1
  Selector3/1 -> dq/1
  abc/dq1/1 -> Selector3/1
  Mux2/1 -> abc/dq1/2
  theta/1 -> Trigonometric Function3/1, Trigonometric Function2/1
  Trigonometric Function2/1 -> Mux2/1
  Trigonometric Function3/1 -> Mux2/2

== system RT_IGBT/SM_SWF/Rec_VQcontrol1/pqctrl/dq ctlr/abc_dq1 ==
  abc : Inport
  theta : Inport  Port=2
  Mux2 : Mux  Inputs=2
  Selector3 : Selector  InputPortWidth=3  IndexOptions=Index vector (dialog)  Indices=[1 2]  OutputSizes=1
  Trigonometric Function2 : Trigonometry
  Trigonometric Function3 : Trigonometry  Operator=cos
  abc/dq1 : powerlib_extras/Measurements/abc_to_dq0 Transformation
  dq : Outport  VectorParamsAs1DForOutWhenUnconnected=off
  wires:
  Trigonometric Function3/1 -> Mux2/2
  Trigonometric Function2/1 -> Mux2/1
  theta/1 -> Trigonometric Function2/1, Trigonometric Function3/1
  Mux2/1 -> abc/dq1/2
  abc/dq1/1 -> Selector3/1
  Selector3/1 -> dq/1
  abc/1 -> abc/dq1/1

== system RT_IGBT/SM_SWF/Rec_VQcontrol1/pqctrl/dq ctlr/measure ==
  note: this is to validate Rxpu and Lxpu which make PI(error) almost zero,
      | i.e. the delay is properly set
      |
      | or to calculate Rxpu and Lxpu which make PI(error) zero
      | when input are in steady state
      |
      | when change the P,Q ref,
      | the results should be same if delay is properly cancelled
  A=X-V : Inport
  Idqref : Inport  Port=2
  Display1 : Display
      settings: Decimation=200
  Fcn7 : Fcn  Expr=(u[2] *u[3]-u[1]*u[4])/(u[3]^2+u[4]^2)
  Fcn8 : Fcn  Expr=(u[1] *u[3]+u[2]*u[4])/(u[3]^2+u[4]^2)
  Mux3 : Mux  Inputs=2
  Mux4 : Mux  Inputs=2
  wires:
  Mux3/1 -> Fcn8/1, Fcn7/1
  Fcn8/1 -> Mux4/1  "Rxpu"
  Fcn7/1 -> Mux4/2  "Lxpu"
  A=X-V/1 -> Mux3/1
  Idqref/1 -> Mux3/2
  Mux4/1 -> Display1/1
